simulink model "flattening_3_test"  (Simulink 7.2)
settings: Solver=ode45  StartTime=0.0  StopTime=10.0  RelTol=1e-3
settings Model: Creator=arnaud  LastModifiedBy=arnaud

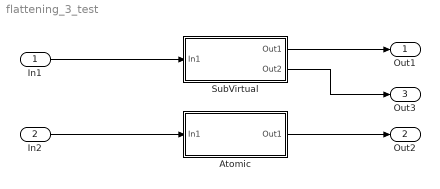
== system flattening_3_test ==
  In1 : Inport  OutDataType=sfix(16)  OutScaling=2^0
  In2 : Inport  Port=2  OutDataType=sfix(16)  OutScaling=2^0
  Atomic : Subsystem  TreatAsAtomicUnit=on
  SubVirtual : Subsystem
  Out1 : Outport  OutDataType=sfix(16)  OutScaling=2^0
  Out2 : Outport  Port=2  OutDataType=sfix(16)  OutScaling=2^0
  Out3 : Outport  Port=3  OutDataType=sfix(16)  OutScaling=2^0
  wires:
  SubVirtual/1(Out1) -> Out1/1
  Atomic/1(Out1) -> Out2/1
  In1/1 -> SubVirtual/1(In1)
  In2/1 -> Atomic/1(In1)
  SubVirtual/2(Out2) -> Out3/1

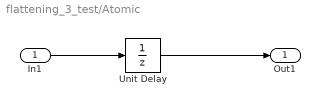
== system flattening_3_test/Atomic ==
  In1 : Inport  OutDataType=sfix(16)  OutScaling=2^0
  Unit Delay : UnitDelay
  Out1 : Outport  OutDataType=sfix(16)  OutScaling=2^0
  wires:
  In1/1 -> Unit Delay/1
  Unit Delay/1 -> Out1/1

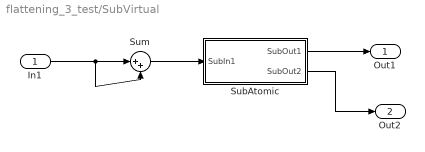
== system flattening_3_test/SubVirtual ==
  In1 : Inport  OutDataType=sfix(16)  OutScaling=2^0
  SubAtomic : Subsystem  TreatAsAtomicUnit=on
  Sum : Sum  Inputs=|++  OutDataType=sfix(16)  OutScaling=2^0
  Out1 : Outport  OutDataType=sfix(16)  OutScaling=2^0
  Out2 : Outport  Port=2  OutDataType=sfix(16)  OutScaling=2^0
  wires:
  SubAtomic/1(SubOut1) -> Out1/1
  Sum/1 -> SubAtomic/1(SubIn1)
  In1/1 -> Sum/1, Sum/2
  SubAtomic/2(SubOut2) -> Out2/1

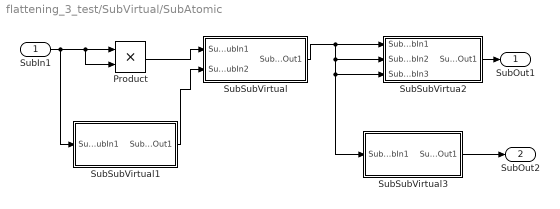
== system flattening_3_test/SubVirtual/SubAtomic ==
  SubIn1 : Inport  OutDataType=sfix(16)  OutScaling=2^0
  Product : Product  OutDataType=sfix(16)  OutScaling=2^0  RndMeth=Zero
  SubSubVirtua2 : Subsystem
  SubSubVirtual : Subsystem
  SubSubVirtual1 : Subsystem
  SubSubVirtual3 : Subsystem
  SubOut1 : Outport  OutDataType=sfix(16)  OutScaling=2^0
  SubOut2 : Outport  Port=2  OutDataType=sfix(16)  OutScaling=2^0
  wires:
  SubSubVirtual/1(SubSubOut1) -> SubSubVirtua2/1(SubSubIn1), SubSubVirtua2/2(SubSubIn2), SubSubVirtua2/3(SubSubIn3), SubSubVirtual3/1(SubSubIn1)
  Product/1 -> SubSubVirtual/1(SubSubIn1)
  SubIn1/1 -> Product/1, Product/2, SubSubVirtual1/1(SubSubIn1)
  SubSubVirtual1/1(SubSubOut1) -> SubSubVirtual/2(SubSubIn2)
  SubSubVirtua2/1(SubSubOut1) -> SubOut1/1
  SubSubVirtual3/1(SubSubOut1) -> SubOut2/1

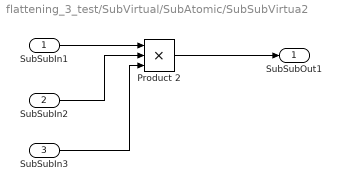
== system flattening_3_test/SubVirtual/SubAtomic/SubSubVirtua2 ==
  SubSubIn1 : Inport  OutDataType=sfix(16)  OutScaling=2^0
  SubSubIn2 : Inport  Port=2  OutDataType=sfix(16)  OutScaling=2^0
  SubSubIn3 : Inport  Port=3  OutDataType=sfix(16)  OutScaling=2^0
  Product 2 : Product  Inputs=3  OutDataType=sfix(16)  OutScaling=2^0  RndMeth=Zero
  SubSubOut1 : Outport  OutDataType=sfix(16)  OutScaling=2^0
  wires:
  SubSubIn1/1 -> Product 2/1
  Product 2/1 -> SubSubOut1/1
  SubSubIn2/1 -> Product 2/2
  SubSubIn3/1 -> Product 2/3

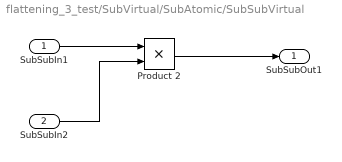
== system flattening_3_test/SubVirtual/SubAtomic/SubSubVirtual ==
  SubSubIn1 : Inport  OutDataType=sfix(16)  OutScaling=2^0
  SubSubIn2 : Inport  Port=2  OutDataType=sfix(16)  OutScaling=2^0
  Product 2 : Product  OutDataType=sfix(16)  OutScaling=2^0  RndMeth=Zero
  SubSubOut1 : Outport  OutDataType=sfix(16)  OutScaling=2^0
  wires:
  SubSubIn1/1 -> Product 2/1
  Product 2/1 -> SubSubOut1/1
  SubSubIn2/1 -> Product 2/2

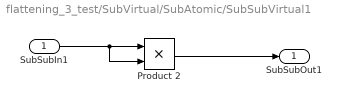
== system flattening_3_test/SubVirtual/SubAtomic/SubSubVirtual1 ==
  SubSubIn1 : Inport  OutDataType=sfix(16)  OutScaling=2^0
  Product 2 : Product  OutDataType=sfix(16)  OutScaling=2^0  RndMeth=Zero
  SubSubOut1 : Outport  OutDataType=sfix(16)  OutScaling=2^0
  wires:
  SubSubIn1/1 -> Product 2/1, Product 2/2
  Product 2/1 -> SubSubOut1/1

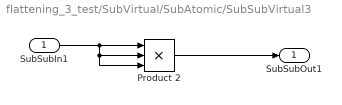
== system flattening_3_test/SubVirtual/SubAtomic/SubSubVirtual3 ==
  SubSubIn1 : Inport  OutDataType=sfix(16)  OutScaling=2^0
  Product 2 : Product  Inputs=3  OutDataType=sfix(16)  OutScaling=2^0  RndMeth=Zero
  SubSubOut1 : Outport  OutDataType=sfix(16)  OutScaling=2^0
  wires:
  SubSubIn1/1 -> Product 2/1, Product 2/2, Product 2/3
  Product 2/1 -> SubSubOut1/1
